simulink model "GA_MPC_sim"  (R2019a)
settings: Solver=VariableStepAuto  StartTime=0.0  StopTime=17  RelTol=1e-3
undefined symbols (not defined in the file or in its folder): param, sigbuilder_block
libraries: mpclib x1
settings Model: Creator=ICS  LastModifiedBy=ICS

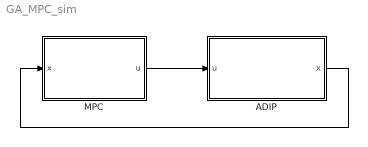
== system GA_MPC_sim ==
  ADIP : Subsystem
  MPC : Subsystem
  wires:
  MPC/1(u) -> ADIP/1(u)
  ADIP/1(x) -> MPC/1(x)

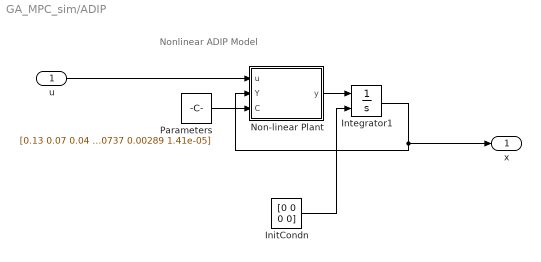
== system GA_MPC_sim/ADIP ==
  note: Nonlinear ADIP Model
  u : Inport
  InitCondn : Constant  Value=[0 0 0 0]
  Integrator1 : Integrator  InitialConditionSource=external  InitialCondition=param.theta0
  "Non-linear Plant " : MATLAB Function  TreatAsAtomicUnit=on
  Parameters : Constant  Value=[0.13 0.07 0.04 0.154 0.186 -9.81 0.0003 0.000202 0.00015814 0.000737 0.00289 1.41e-05]
  x : Outport
  wires:
  "Non-linear Plant "/1(y) -> Integrator1/1
  Integrator1/1 -> x/1, "Non-linear Plant "/2(Y)
  u/1 -> "Non-linear Plant "/1(u)
  Parameters/1 -> "Non-linear Plant "/3(C)
  InitCondn/1 -> Integrator1/2

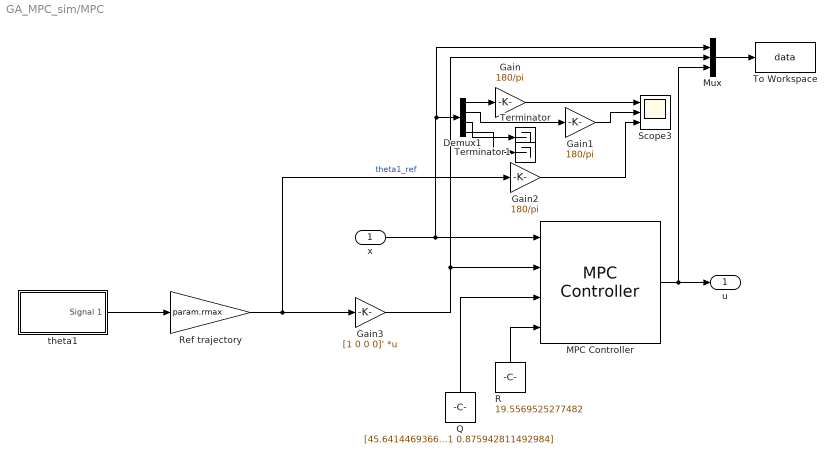
== system GA_MPC_sim/MPC ==
  x : Inport
  Demux1 : Demux
  Gain : Gain  Gain=180/pi
  Gain1 : Gain  Gain=180/pi
  Gain2 : Gain  Gain=180/pi
  Gain3 : Gain  Gain=[1 0 0 0]'  Multiplication=Matrix(K*u)
  MPC Controller : mpclib/MPC Controller  SCDEnableBlockLinearizationSpecification=on  mpcobj=MPCobj  is_multiple=0  enable_value=0  return_u0=off  updateMPCinCallerWorkspace=on  md_inport=off  mv_inport=off  uref_inport=off  return_cost=off  return_mvseq=off  return_qpstatus=off  return_xseq=off  return_state=off  return_ovseq=off  state_inport=off  umin_inport=off  umax_inport=off  ymin_inport=off  ymax_inport=off  cc_inport=off  ywt_inport=on  uwt_inport=on  duwt_inport=off  rhoeps_inport=off  pm_inport=off  MaximumP=10  HorizonChoice=FixedHorizon  n_ts=0.01  n_p=100  n_mv=1  n_md=0  n_ud=0  n_mo=4  n_uo=0  BlockDataType=double  SampleTimeInherited=off  switch_inport=off
      settings: SourceProductName=MATLAB Runtime - Model Predictive Control Toolbox Addin  SourceProductBaseCode=Missing
  Mux : Mux  Inputs=3
  Q : Constant  Value=[45.6414469366635 78.2425160799863 5.1077156417211 0.875942811492984]
  R : Constant  Value=19.5569525277482
  Ref trajectory : Gain  Gain=param.rmax
  Scope3 : Scope  NumInputPorts=3
  Terminator : Terminator
  Terminator1 : Terminator
  To Workspace : ToWorkspace  VariableName=data  SampleTime=-1
  theta1 : Subsystem  Tag=STV Subsys  LoadFcn=sigbuilder_block('load');  StartFcn=sigbuilder_block('start');  StopFcn=sigbuilder_block('stop');  ClipboardFcn=sigbuilder_block('clipboard');  mask(Sigbuilder block){tuvar=[0:10]}
      mask help: Simulink:masks:SigbuilderBlock_MD
      mask init:
      | if ~strcmp(get_param(bdroot(gcbh),'SimulationStatus'),'stopped') tuvar = sigbuilder_block('maskInit'); end
      settings: CopyFcn=sigbuilder_block('copy');  DeleteFcn=sigbuilder_block('delete');  ModelCloseFcn=sigbuilder_block('modelClose');  PreSaveFcn=sigbuilder_block('preSave');  PauseFcn=sigbuilder_block('pause');  ContinueFcn=sigbuilder_block('continue');  NameChangeFcn=sigbuilder_block('namechange');  OpenFcn=sigbuilder_block('open',[5.5 30 1909 958 ]);  CloseFcn=sigbuilder_block('close');
      mask Display: plot(0, 0, 100, 100,[2, 2, 32, 32, 2], [68, 8, 8, 68, 68],[32, 2], [38, 38], [32, 19, 2],[53, 60, 44], [32, 17, 17, 2],[16, 16, 31, 31]);txt = getActiveGroup(gcbh);text(2, 100, txt,'verticalAlignment', 'top');
  u : Outport
  wires:
  Ref trajectory/1 -> Gain2/1, Gain3/1  "theta1_ref"
  MPC Controller/1 -> Mux/3, u/1
  x/1 -> Mux/1, Demux1/1, MPC Controller/1
  Demux1/1 -> Gain/1
  Demux1/2 -> Gain1/1
  Gain/1 -> Scope3/1
  Gain1/1 -> Scope3/2
  Gain2/1 -> Scope3/3
  Mux/1 -> To Workspace/1
  Demux1/3 -> Terminator/1
  Demux1/4 -> Terminator1/1
  Q/1 -> MPC Controller/3
  R/1 -> MPC Controller/4
  theta1/1(Signal 1) -> Ref trajectory/1
  Gain3/1 -> Mux/2, MPC Controller/2

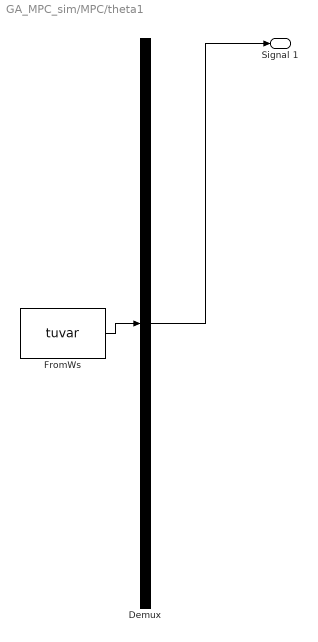
== system GA_MPC_sim/MPC/theta1 ==
  Demux : Demux  Tag=STV Demux  Outputs=1
  FromWs : FromWorkspace  Tag=STV FromWs  VariableName=tuvar  SampleTime=0
      SigBuilderData=|
      | common.afterFinalStr = 'Extrapolate'
      | common.sampleTime = 0
      | dataSet.timeRange = [0 50]
      | dataSet.name = 'Group 1'
      | sbobj.Groups.Name = 'Group 1'
      | sbobj.Groups.Signals.Name = 'Signal 1'
      | sbobj.Groups.Signals.XData = [0 2 5 6.5 10.5 12 15 50]
      | sbobj.Groups.Signals.YData = [0 0 1 1 -1 -1 0 0]
      | sbobj.Groups.TimeRange = [0 50]
  Signal 1 : Outport  Tag=STV Outport
  wires:
  Demux/1 -> Signal 1/1
  FromWs/1 -> Demux/1

== matlab function GA_MPC_sim/ADIP/Non-linear Plant  ==
  data: u input; Y input; y output; C input
function y = fcn(u,Y,C)
m1=C(1); % Mass of arm
m2=C(2); % Mass of pendulum
mh = C(3); % Mass of Hinge
l1  = C(4); % Length of arm
l2 = C(5); % Length of pendulum
g_ = C(6);
J_arm = C(7);
J_pend = C(8);
J_motor = C(9);
J_sensor = C(10);
fv1 = C(11);
fv2 = C(12);

y1 = Y(1);  % actual theta1          
y2 = Y(2);  % actual theta2
y3 = Y(3);  % actual theta1d
y4 = Y(4);  % actual theta2d

dy1 = y3;
dy2 = y4;
dy3 =-(2*(8*J_pend*fv1*y3 - 2*l2^2*m2*u - 8*J_pend*u + 2*fv1*l2^2*m2*y3 + l1^2*l2^2*m2^2*y3^2*sin(2*y1 - 2*y2) + l1*l2^3*m2^2*y4^2*sin(y1 - y2) + g_*l1*l2^2*m2^2*sin(y1) + 4*J_pend*g_*l1*m1*sin(y1) + 8*J_pend*g_*l1*m2*sin(y1) + 8*J_pend*g_*l1*mh*sin(y1) + g_*l1*l2^2*m2^2*sin(y1 - 2*y2) - 4*fv2*l1*l2*m2*y4*cos(y1 - y2) + g_*l1*l2^2*m1*m2*sin(y1) + 2*g_*l1*l2^2*m2*mh*sin(y1) + 4*J_pend*l1*l2*m2*y4^2*sin(y1 - y2)))/(16*J_arm*J_pend + 16*J_motor*J_pend + 16*J_pend*J_sensor + 4*l1^2*l2^2*m2^2 + 4*J_arm*l2^2*m2 + 4*J_motor*l2^2*m2 + 4*J_pend*l1^2*m1 + 16*J_pend*l1^2*m2 + 4*J_sensor*l2^2*m2 - 4*l1^2*l2^2*m2^2*cos(y1 - y2)^2 + l1^2*l2^2*m1*m2);
dy4 =(2*(l1^2*l2^2*m2^2*y4^2*sin(2*y1 - 2*y2) - 8*J_motor*fv2*y4 - 8*J_sensor*fv2*y4 - 2*fv2*l1^2*m1*y4 - 8*fv2*l1^2*m2*y4 - 8*J_arm*fv2*y4 - 4*l1*l2*m2*u*cos(y1 - y2) + 2*g_*l1^2*l2*m2^2*sin(2*y1 - y2) + 4*l1^3*l2*m2^2*y3^2*sin(y1 - y2) - 2*g_*l1^2*l2*m2^2*sin(y2) - 4*J_arm*g_*l2*m2*sin(y2) - 4*J_motor*g_*l2*m2*sin(y2) - 4*J_sensor*g_*l2*m2*sin(y2) + g_*l1^2*l2*m1*m2*sin(2*y1 - y2) + 2*g_*l1^2*l2*m2*mh*sin(2*y1 - y2) + l1^3*l2*m1*m2*y3^2*sin(y1 - y2) + 4*fv1*l1*l2*m2*y3*cos(y1 - y2) + 2*g_*l1^2*l2*m2*mh*sin(y2) + 4*J_arm*l1*l2*m2*y3^2*sin(y1 - y2) + 4*J_motor*l1*l2*m2*y3^2*sin(y1 - y2) + 4*J_sensor*l1*l2*m2*y3^2*sin(y1 - y2)))/(16*J_arm*J_pend + 16*J_motor*J_pend + 16*J_pend*J_sensor + 2*l1^2*l2^2*m2^2 + 4*J_arm*l2^2*m2 + 4*J_motor*l2^2*m2 + 4*J_pend*l1^2*m1 + 16*J_pend*l1^2*m2 + 4*J_sensor*l2^2*m2 - 2*l1^2*l2^2*m2^2*cos(2*y1 - 2*y2) + l1^2*l2^2*m1*m2);
y = [dy1 dy2 dy3 dy4]';
